simulink model "Huang_Isoherranen_Mechanistic_Kidney_Model"  (R2017b)
settings: Solver=VariableStepAuto  StartTime=0.0  StopTime=Tfinish  RelTol=1e-3  EnableMultiTasking=on
values from neighbouring files (symbols this model uses):
  alpha_1 = 1    [Huang_Isoherranen_Mechanistic_Kidney_Model_Example_Code.m]
  alpha_10 = 1    [Huang_Isoherranen_Mechanistic_Kidney_Model_Example_Code.m]
  alpha_11 = 1    [Huang_Isoherranen_Mechanistic_Kidney_Model_Example_Code.m]
  alpha_2 = 1    [Huang_Isoherranen_Mechanistic_Kidney_Model_Example_Code.m]
  alpha_3 = 1    [Huang_Isoherranen_Mechanistic_Kidney_Model_Example_Code.m]
  alpha_4 = 1    [Huang_Isoherranen_Mechanistic_Kidney_Model_Example_Code.m]
  alpha_5 = 1    [Huang_Isoherranen_Mechanistic_Kidney_Model_Example_Code.m]
  alpha_6 = 1    [Huang_Isoherranen_Mechanistic_Kidney_Model_Example_Code.m]
  alpha_7 = 1    [Huang_Isoherranen_Mechanistic_Kidney_Model_Example_Code.m]
  alpha_8 = 1    [Huang_Isoherranen_Mechanistic_Kidney_Model_Example_Code.m]
  alpha_9 = 1    [Huang_Isoherranen_Mechanistic_Kidney_Model_Example_Code.m]
  beta = 1    [Huang_Isoherranen_Mechanistic_Kidney_Model_Example_Code.m]
  BP0 = 1    [Huang_Isoherranen_Mechanistic_Kidney_Model_Example_Code.m]
  CL_api_reabs = 0    [Huang_Isoherranen_Mechanistic_Kidney_Model_Example_Code.m]
  CL_BC = 0    [Huang_Isoherranen_Mechanistic_Kidney_Model_Example_Code.m]
  CL_bsl_reabs = 0    [Huang_Isoherranen_Mechanistic_Kidney_Model_Example_Code.m]
  CL_CT = 0    [Huang_Isoherranen_Mechanistic_Kidney_Model_Example_Code.m]
  CL_kidney_intrinsic = 0    [Huang_Isoherranen_Mechanistic_Kidney_Model_Example_Code.m]
  CL_PD_CD = S_CD * Papp    (= 0.01608)    [Huang_Isoherranen_Mechanistic_Kidney_Model_Example_Code.m]
  CL_PD_DS = S_DT * Papp    (= 0.3744)    [Huang_Isoherranen_Mechanistic_Kidney_Model_Example_Code.m]
  CL_PD_LH = S_HT * Papp    (= 0.1464)    [Huang_Isoherranen_Mechanistic_Kidney_Model_Example_Code.m]
  CL_PD_PX_apical = S_PT * Papp    (= 14.6568)    [Huang_Isoherranen_Mechanistic_Kidney_Model_Example_Code.m]
  CL_PD_PX_basolateral = S_PT/30 * Papp    (= 0.48856)    [Huang_Isoherranen_Mechanistic_Kidney_Model_Example_Code.m]
  CLh = 0    [Huang_Isoherranen_Mechanistic_Kidney_Model_Example_Code.m]
  fu0 = 1    [Huang_Isoherranen_Mechanistic_Kidney_Model_Example_Code.m]
  fu_k = fu0    (= 1)    [Huang_Isoherranen_Mechanistic_Kidney_Model_Example_Code.m]
  gamma = 1    [Huang_Isoherranen_Mechanistic_Kidney_Model_Example_Code.m]
  Infusion_length = 240    [Huang_Isoherranen_Mechanistic_Kidney_Model_Example_Code.m]
  IR = 1    [Huang_Isoherranen_Mechanistic_Kidney_Model_Example_Code.m]
  ivbolusDose1 = 0    [Huang_Isoherranen_Mechanistic_Kidney_Model_Example_Code.m]
  ivT1 = 0    [Huang_Isoherranen_Mechanistic_Kidney_Model_Example_Code.m]
  Q_connectingtubule = 11    [Huang_Isoherranen_Mechanistic_Kidney_Model_Example_Code.m]
  Q_corticalCD = 7    [Huang_Isoherranen_Mechanistic_Kidney_Model_Example_Code.m]
  Q_GFR = 7.2    [Huang_Isoherranen_Mechanistic_Kidney_Model_Example_Code.m]
  Q_initialCD = 9    [Huang_Isoherranen_Mechanistic_Kidney_Model_Example_Code.m]
  Q_kidney0 = 60    [Huang_Isoherranen_Mechanistic_Kidney_Model_Example_Code.m]
  Q_medullaryCD = 5    [Huang_Isoherranen_Mechanistic_Kidney_Model_Example_Code.m]
  Q_papillary = 3    [Huang_Isoherranen_Mechanistic_Kidney_Model_Example_Code.m]
  Q_urine = 1    [Huang_Isoherranen_Mechanistic_Kidney_Model_Example_Code.m]
  Qc0 = 330    [Huang_Isoherranen_Mechanistic_Kidney_Model_Example_Code.m]
  Tstart_infusion = 0    [Huang_Isoherranen_Mechanistic_Kidney_Model_Example_Code.m]
  V_CDB = 0.237    [Huang_Isoherranen_Mechanistic_Kidney_Model_Example_Code.m]
  V_CDC = 0.237    [Huang_Isoherranen_Mechanistic_Kidney_Model_Example_Code.m]
  V_CDT = 0.237    [Huang_Isoherranen_Mechanistic_Kidney_Model_Example_Code.m]
  V_DB = 0.0194    [Huang_Isoherranen_Mechanistic_Kidney_Model_Example_Code.m]
  V_DC = 0.0194    [Huang_Isoherranen_Mechanistic_Kidney_Model_Example_Code.m]
  V_DT = 0.0194    [Huang_Isoherranen_Mechanistic_Kidney_Model_Example_Code.m]
  V_HB = 0.0027    [Huang_Isoherranen_Mechanistic_Kidney_Model_Example_Code.m]
  V_HC = 0.0027    [Huang_Isoherranen_Mechanistic_Kidney_Model_Example_Code.m]
  V_HT = 0.0027    [Huang_Isoherranen_Mechanistic_Kidney_Model_Example_Code.m]
  V_PB = 0.0305    [Huang_Isoherranen_Mechanistic_Kidney_Model_Example_Code.m]
  V_PC = 0.0305    [Huang_Isoherranen_Mechanistic_Kidney_Model_Example_Code.m]
  V_PT = 0.0305    [Huang_Isoherranen_Mechanistic_Kidney_Model_Example_Code.m]
  V_ven0 = 42    [Huang_Isoherranen_Mechanistic_Kidney_Model_Example_Code.m]
libraries: simulink x3, dspmathops x1
(part 2 of 2)

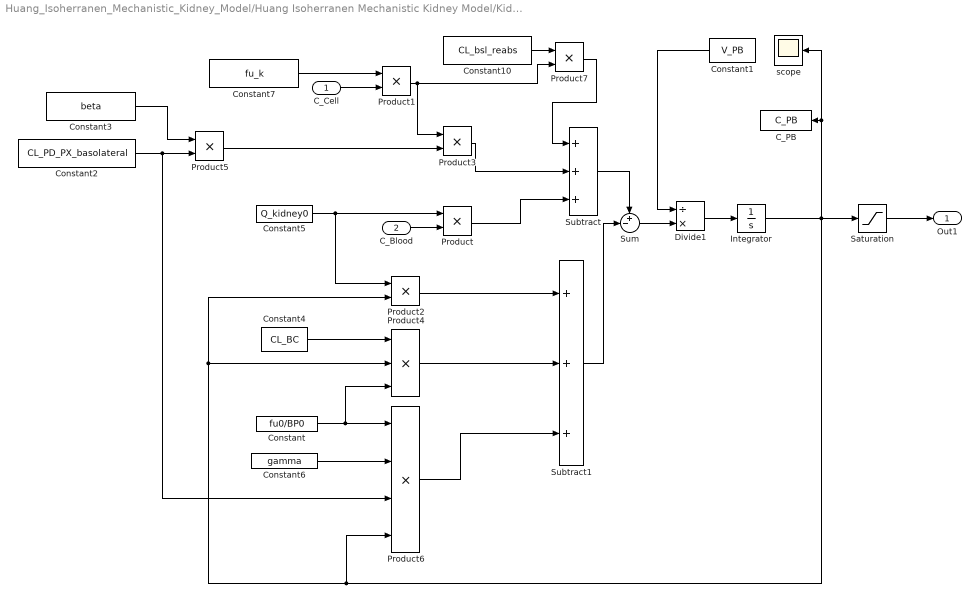
== system Huang_Isoherranen_Mechanistic_Kidney_Model/Huang Isoherranen Mechanistic Kidney Model/Kidney/Proximal blood ==
  C_Cell : Inport
  C_Blood : Inport  Port=2
  C_PB : ToWorkspace  VariableName=C_PB  SampleTime=-1
  Constant : Constant  Value=fu0/BP0
  Constant1 : Constant  Value=V_PB
  Constant10 : Constant  Value=CL_bsl_reabs
  Constant2 : Constant  Value=CL_PD_PX_basolateral
  Constant3 : Constant  Value=beta
  Constant4 : Constant  Value=CL_BC
  Constant5 : Constant  Value=Q_kidney0
  Constant6 : Constant  Value=gamma
  Constant7 : Constant  Value=fu_k
  Divide1 : Product  Inputs=/*
  Integrator : Integrator
  Product{,1..3,5,7} (6 alike) : Product  RndMeth=Zero
  Product4 : Product  Inputs=3  RndMeth=Zero
  Product6 : Product  Inputs=4  RndMeth=Zero
  Saturation : Saturate  UpperLimit=1000000000  LowerLimit=0
  Subtract : Sum  Inputs=+++
  Subtract1 : Sum  Inputs=+++
  Sum : Sum  Inputs=+-|
  scope : Scope
  Out1 : Outport
  wires:
  Integrator/1 -> Product6/4, Product2/2, Product4/2, Saturation/1, scope/1, C_PB/1
  Sum/1 -> Divide1/2
  Saturation/1 -> Out1/1
  Constant7/1 -> Product1/1
  Product1/1 -> Product3/1, Product7/2
  Constant5/1 -> Product2/1, Product/1
  Product3/1 -> Subtract/2
  Product/1 -> Subtract/3
  Constant1/1 -> Divide1/1
  Subtract/1 -> Sum/1
  Divide1/1 -> Integrator/1
  Constant3/1 -> Product5/1
  Constant2/1 -> Product6/3, Product5/2
  Product5/1 -> Product3/2
  Subtract1/1 -> Sum/2
  C_Cell/1 -> Product1/2
  C_Blood/1 -> Product/2
  Constant/1 -> Product4/3, Product6/1
  Product2/1 -> Subtract1/1
  Constant6/1 -> Product6/2
  Product6/1 -> Subtract1/3
  Constant4/1 -> Product4/1
  Product4/1 -> Subtract1/2
  Constant10/1 -> Product7/1
  Product7/1 -> Subtract/1

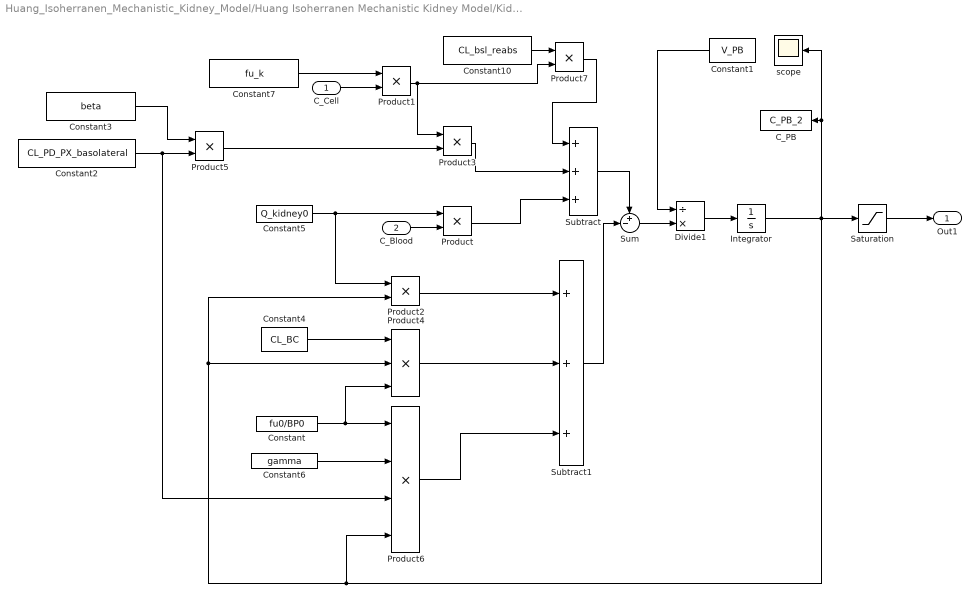
== system Huang_Isoherranen_Mechanistic_Kidney_Model/Huang Isoherranen Mechanistic Kidney Model/Kidney/Proximal blood1 ==
  C_Cell : Inport
  C_Blood : Inport  Port=2
  C_PB : ToWorkspace  VariableName=C_PB_2  SampleTime=-1
  Constant : Constant  Value=fu0/BP0
  Constant1 : Constant  Value=V_PB
  Constant10 : Constant  Value=CL_bsl_reabs
  Constant2 : Constant  Value=CL_PD_PX_basolateral
  Constant3 : Constant  Value=beta
  Constant4 : Constant  Value=CL_BC
  Constant5 : Constant  Value=Q_kidney0
  Constant6 : Constant  Value=gamma
  Constant7 : Constant  Value=fu_k
  Divide1 : Product  Inputs=/*
  Integrator : Integrator
  Product{,1..3,5,7} (6 alike) : Product  RndMeth=Zero
  Product4 : Product  Inputs=3  RndMeth=Zero
  Product6 : Product  Inputs=4  RndMeth=Zero
  Saturation : Saturate  UpperLimit=1000000000  LowerLimit=0
  Subtract : Sum  Inputs=+++
  Subtract1 : Sum  Inputs=+++
  Sum : Sum  Inputs=+-|
  scope : Scope
  Out1 : Outport
  wires:
  Integrator/1 -> Product6/4, Product2/2, Product4/2, Saturation/1, scope/1, C_PB/1
  Sum/1 -> Divide1/2
  Saturation/1 -> Out1/1
  Constant7/1 -> Product1/1
  Product1/1 -> Product3/1, Product7/2
  Constant5/1 -> Product2/1, Product/1
  Product3/1 -> Subtract/2
  Product/1 -> Subtract/3
  Constant1/1 -> Divide1/1
  Subtract/1 -> Sum/1
  Divide1/1 -> Integrator/1
  Constant3/1 -> Product5/1
  Constant2/1 -> Product6/3, Product5/2
  Product5/1 -> Product3/2
  Subtract1/1 -> Sum/2
  C_Cell/1 -> Product1/2
  C_Blood/1 -> Product/2
  Constant/1 -> Product4/3, Product6/1
  Product2/1 -> Subtract1/1
  Constant6/1 -> Product6/2
  Product6/1 -> Subtract1/3
  Constant4/1 -> Product4/1
  Product4/1 -> Subtract1/2
  Constant10/1 -> Product7/1
  Product7/1 -> Subtract/1

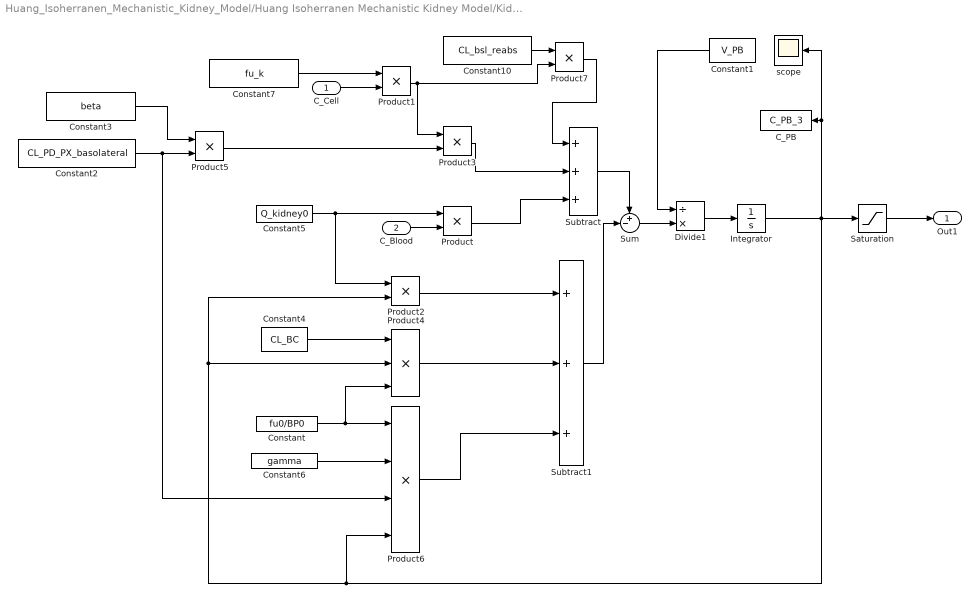
== system Huang_Isoherranen_Mechanistic_Kidney_Model/Huang Isoherranen Mechanistic Kidney Model/Kidney/Proximal blood2 ==
  C_Cell : Inport
  C_Blood : Inport  Port=2
  C_PB : ToWorkspace  VariableName=C_PB_3  SampleTime=-1
  Constant : Constant  Value=fu0/BP0
  Constant1 : Constant  Value=V_PB
  Constant10 : Constant  Value=CL_bsl_reabs
  Constant2 : Constant  Value=CL_PD_PX_basolateral
  Constant3 : Constant  Value=beta
  Constant4 : Constant  Value=CL_BC
  Constant5 : Constant  Value=Q_kidney0
  Constant6 : Constant  Value=gamma
  Constant7 : Constant  Value=fu_k
  Divide1 : Product  Inputs=/*
  Integrator : Integrator
  Product{,1..3,5,7} (6 alike) : Product  RndMeth=Zero
  Product4 : Product  Inputs=3  RndMeth=Zero
  Product6 : Product  Inputs=4  RndMeth=Zero
  Saturation : Saturate  UpperLimit=1000000000  LowerLimit=0
  Subtract : Sum  Inputs=+++
  Subtract1 : Sum  Inputs=+++
  Sum : Sum  Inputs=+-|
  scope : Scope
  Out1 : Outport
  wires:
  Integrator/1 -> Product6/4, Product2/2, Product4/2, Saturation/1, scope/1, C_PB/1
  Sum/1 -> Divide1/2
  Saturation/1 -> Out1/1
  Constant7/1 -> Product1/1
  Product1/1 -> Product3/1, Product7/2
  Constant5/1 -> Product2/1, Product/1
  Product3/1 -> Subtract/2
  Product/1 -> Subtract/3
  Constant1/1 -> Divide1/1
  Subtract/1 -> Sum/1
  Divide1/1 -> Integrator/1
  Constant3/1 -> Product5/1
  Constant2/1 -> Product6/3, Product5/2
  Product5/1 -> Product3/2
  Subtract1/1 -> Sum/2
  C_Cell/1 -> Product1/2
  C_Blood/1 -> Product/2
  Constant/1 -> Product4/3, Product6/1
  Product2/1 -> Subtract1/1
  Constant6/1 -> Product6/2
  Product6/1 -> Subtract1/3
  Constant4/1 -> Product4/1
  Product4/1 -> Subtract1/2
  Constant10/1 -> Product7/1
  Product7/1 -> Subtract/1

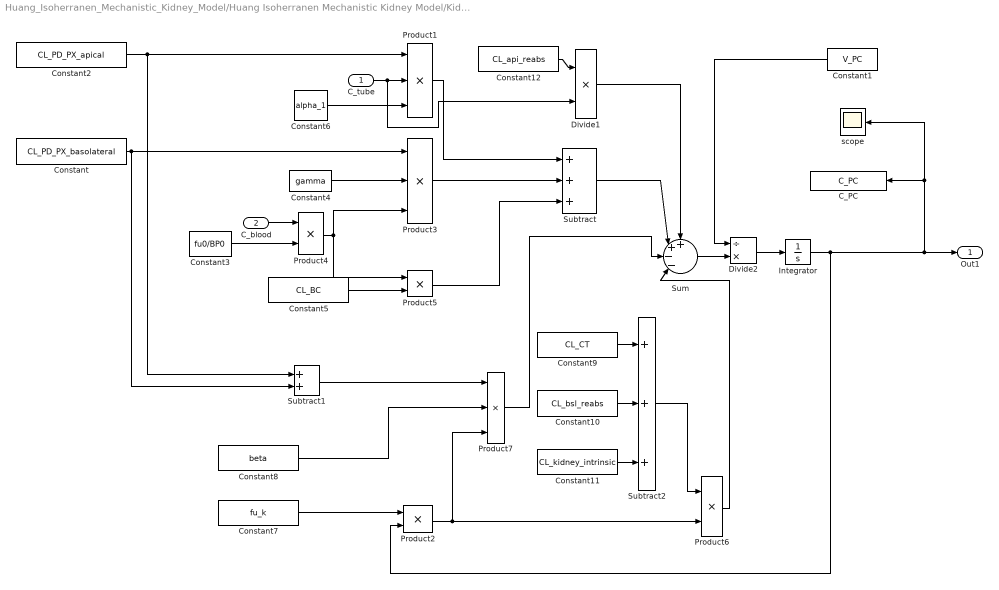
== system Huang_Isoherranen_Mechanistic_Kidney_Model/Huang Isoherranen Mechanistic Kidney Model/Kidney/Proximal cell ==
  C_tube : Inport
  C_blood : Inport  Port=2
  C_PC : ToWorkspace  VariableName=C_PC  SampleTime=-1
  Constant : Constant  Value=CL_PD_PX_basolateral
  Constant1 : Constant  Value=V_PC
  Constant10 : Constant  Value=CL_bsl_reabs
  Constant11 : Constant  Value=CL_kidney_intrinsic
  Constant12 : Constant  Value=CL_api_reabs
  Constant2 : Constant  Value=CL_PD_PX_apical
  Constant3 : Constant  Value=fu0/BP0
  Constant4 : Constant  Value=gamma
  Constant5 : Constant  Value=CL_BC
  Constant6 : Constant  Value=alpha_1
  Constant7 : Constant  Value=fu_k
  Constant8 : Constant  Value=beta
  Constant9 : Constant  Value=CL_CT
  Divide1 : Product  Inputs=**
  Divide2 : Product  Inputs=/*
  Integrator : Integrator
  Product1 : Product  Inputs=3  RndMeth=Zero
  Product{2,4..6} (4 alike) : Product  RndMeth=Zero
  Product3 : Product  Inputs=3  RndMeth=Zero
  Product7 : Product  Inputs=3  RndMeth=Zero
  Subtract : Sum  Inputs=+++
  Subtract1 : Sum
  Subtract2 : Sum  Inputs=+++
  Sum : Sum  Inputs=++--|
  scope : Scope
  Out1 : Outport
  wires:
  Integrator/1 -> Product2/2, Out1/1, scope/1, C_PC/1
  C_tube/1 -> Divide1/2, Product1/2
  Constant2/1 -> Subtract1/1, Product1/1
  Constant4/1 -> Product3/2
  Subtract/1 -> Sum/2
  Product3/1 -> Subtract/2
  C_blood/1 -> Product4/1
  Constant3/1 -> Product4/2
  Product4/1 -> Product5/1, Product3/3
  Constant5/1 -> Product5/2
  Constant6/1 -> Product1/3
  Product5/1 -> Subtract/3
  Product1/1 -> Subtract/1
  Sum/1 -> Divide2/2
  Constant1/1 -> Divide2/1
  Divide2/1 -> Integrator/1
  Product2/1 -> Product6/2, Product7/3
  Constant7/1 -> Product2/1
  Constant8/1 -> Product7/2
  Product6/1 -> Sum/4
  Product7/1 -> Sum/3
  Subtract1/1 -> Product7/1
  Constant/1 -> Subtract1/2, Product3/1
  Constant12/1 -> Divide1/1
  Divide1/1 -> Sum/1
  Constant10/1 -> Subtract2/2
  Subtract2/1 -> Product6/1
  Constant9/1 -> Subtract2/1
  Constant11/1 -> Subtract2/3

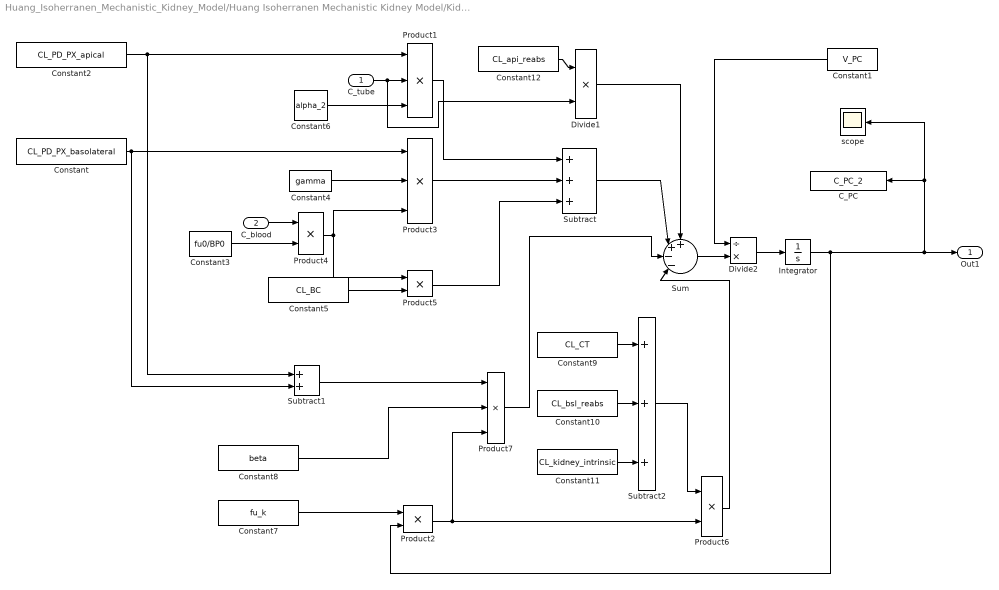
== system Huang_Isoherranen_Mechanistic_Kidney_Model/Huang Isoherranen Mechanistic Kidney Model/Kidney/Proximal cell1 ==
  C_tube : Inport
  C_blood : Inport  Port=2
  C_PC : ToWorkspace  VariableName=C_PC_2  SampleTime=-1
  Constant : Constant  Value=CL_PD_PX_basolateral
  Constant1 : Constant  Value=V_PC
  Constant10 : Constant  Value=CL_bsl_reabs
  Constant11 : Constant  Value=CL_kidney_intrinsic
  Constant12 : Constant  Value=CL_api_reabs
  Constant2 : Constant  Value=CL_PD_PX_apical
  Constant3 : Constant  Value=fu0/BP0
  Constant4 : Constant  Value=gamma
  Constant5 : Constant  Value=CL_BC
  Constant6 : Constant  Value=alpha_2
  Constant7 : Constant  Value=fu_k
  Constant8 : Constant  Value=beta
  Constant9 : Constant  Value=CL_CT
  Divide1 : Product  Inputs=**
  Divide2 : Product  Inputs=/*
  Integrator : Integrator
  Product1 : Product  Inputs=3  RndMeth=Zero
  Product{2,4..6} (4 alike) : Product  RndMeth=Zero
  Product3 : Product  Inputs=3  RndMeth=Zero
  Product7 : Product  Inputs=3  RndMeth=Zero
  Subtract : Sum  Inputs=+++
  Subtract1 : Sum
  Subtract2 : Sum  Inputs=+++
  Sum : Sum  Inputs=++--|
  scope : Scope
  Out1 : Outport
  wires:
  Integrator/1 -> Product2/2, Out1/1, scope/1, C_PC/1
  C_tube/1 -> Divide1/2, Product1/2
  Constant2/1 -> Subtract1/1, Product1/1
  Constant4/1 -> Product3/2
  Subtract/1 -> Sum/2
  Product3/1 -> Subtract/2
  C_blood/1 -> Product4/1
  Constant3/1 -> Product4/2
  Product4/1 -> Product5/1, Product3/3
  Constant5/1 -> Product5/2
  Constant6/1 -> Product1/3
  Product5/1 -> Subtract/3
  Product1/1 -> Subtract/1
  Sum/1 -> Divide2/2
  Constant1/1 -> Divide2/1
  Divide2/1 -> Integrator/1
  Product2/1 -> Product6/2, Product7/3
  Constant7/1 -> Product2/1
  Constant8/1 -> Product7/2
  Product6/1 -> Sum/4
  Product7/1 -> Sum/3
  Subtract1/1 -> Product7/1
  Constant/1 -> Subtract1/2, Product3/1
  Constant12/1 -> Divide1/1
  Divide1/1 -> Sum/1
  Constant10/1 -> Subtract2/2
  Subtract2/1 -> Product6/1
  Constant9/1 -> Subtract2/1
  Constant11/1 -> Subtract2/3

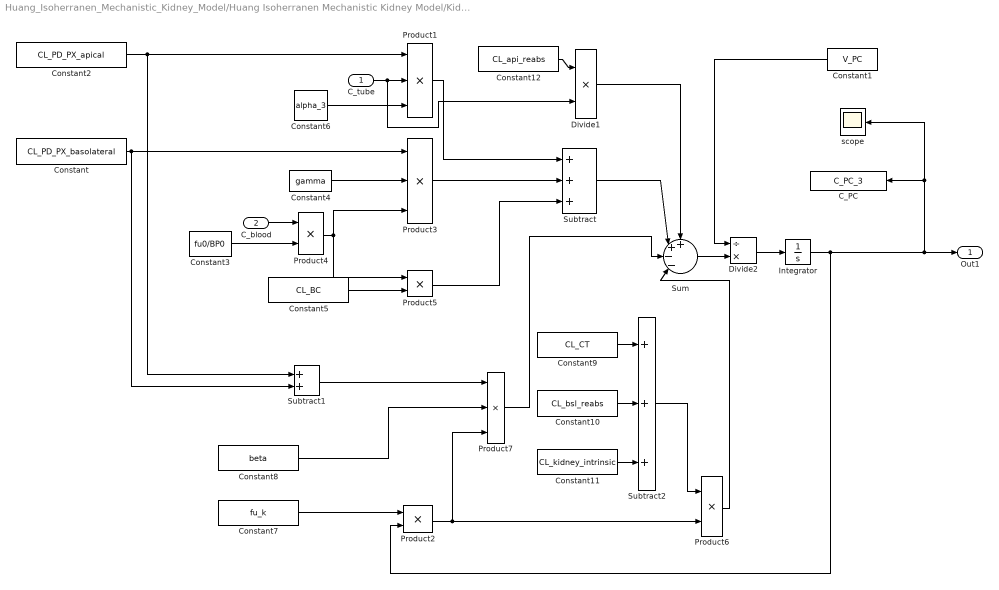
== system Huang_Isoherranen_Mechanistic_Kidney_Model/Huang Isoherranen Mechanistic Kidney Model/Kidney/Proximal cell2 ==
  C_tube : Inport
  C_blood : Inport  Port=2
  C_PC : ToWorkspace  VariableName=C_PC_3  SampleTime=-1
  Constant : Constant  Value=CL_PD_PX_basolateral
  Constant1 : Constant  Value=V_PC
  Constant10 : Constant  Value=CL_bsl_reabs
  Constant11 : Constant  Value=CL_kidney_intrinsic
  Constant12 : Constant  Value=CL_api_reabs
  Constant2 : Constant  Value=CL_PD_PX_apical
  Constant3 : Constant  Value=fu0/BP0
  Constant4 : Constant  Value=gamma
  Constant5 : Constant  Value=CL_BC
  Constant6 : Constant  Value=alpha_3
  Constant7 : Constant  Value=fu_k
  Constant8 : Constant  Value=beta
  Constant9 : Constant  Value=CL_CT
  Divide1 : Product  Inputs=**
  Divide2 : Product  Inputs=/*
  Integrator : Integrator
  Product1 : Product  Inputs=3  RndMeth=Zero
  Product{2,4..6} (4 alike) : Product  RndMeth=Zero
  Product3 : Product  Inputs=3  RndMeth=Zero
  Product7 : Product  Inputs=3  RndMeth=Zero
  Subtract : Sum  Inputs=+++
  Subtract1 : Sum
  Subtract2 : Sum  Inputs=+++
  Sum : Sum  Inputs=++--|
  scope : Scope
  Out1 : Outport
  wires:
  Integrator/1 -> Product2/2, Out1/1, scope/1, C_PC/1
  C_tube/1 -> Divide1/2, Product1/2
  Constant2/1 -> Subtract1/1, Product1/1
  Constant4/1 -> Product3/2
  Subtract/1 -> Sum/2
  Product3/1 -> Subtract/2
  C_blood/1 -> Product4/1
  Constant3/1 -> Product4/2
  Product4/1 -> Product5/1, Product3/3
  Constant5/1 -> Product5/2
  Constant6/1 -> Product1/3
  Product5/1 -> Subtract/3
  Product1/1 -> Subtract/1
  Sum/1 -> Divide2/2
  Constant1/1 -> Divide2/1
  Divide2/1 -> Integrator/1
  Product2/1 -> Product6/2, Product7/3
  Constant7/1 -> Product2/1
  Constant8/1 -> Product7/2
  Product6/1 -> Sum/4
  Product7/1 -> Sum/3
  Subtract1/1 -> Product7/1
  Constant/1 -> Subtract1/2, Product3/1
  Constant12/1 -> Divide1/1
  Divide1/1 -> Sum/1
  Constant10/1 -> Subtract2/2
  Subtract2/1 -> Product6/1
  Constant9/1 -> Subtract2/1
  Constant11/1 -> Subtract2/3

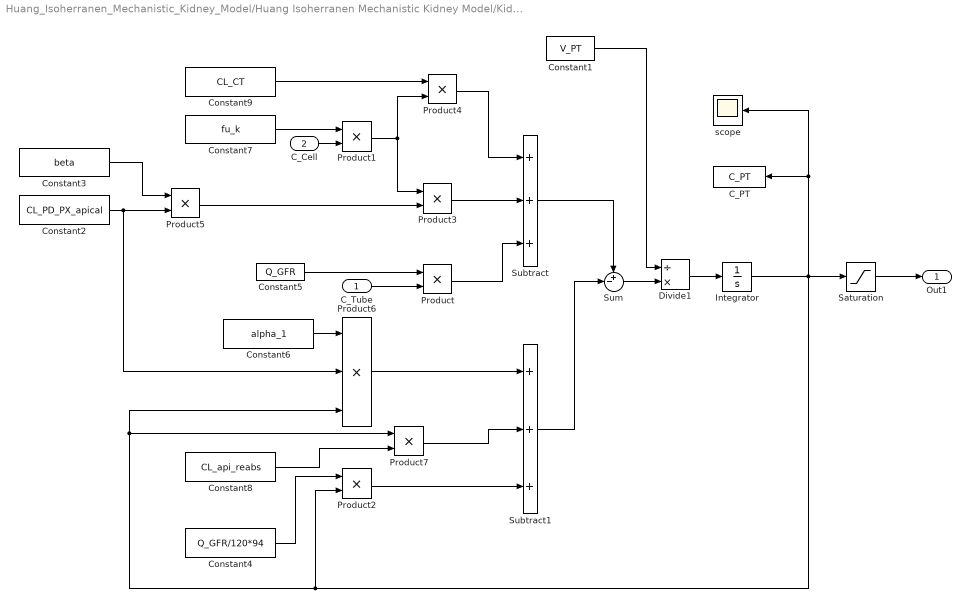
== system Huang_Isoherranen_Mechanistic_Kidney_Model/Huang Isoherranen Mechanistic Kidney Model/Kidney/Proximal tube ==
  C_Tube : Inport
  C_Cell : Inport  Port=2
  C_PT : ToWorkspace  VariableName=C_PT  SampleTime=-1
  Constant1 : Constant  Value=V_PT
  Constant2 : Constant  Value=CL_PD_PX_apical
  Constant3 : Constant  Value=beta
  Constant4 : Constant  Value=Q_GFR/120*94
  Constant5 : Constant  Value=Q_GFR
  Constant6 : Constant  Value=alpha_1
  Constant7 : Constant  Value=fu_k
  Constant8 : Constant  Value=CL_api_reabs
  Constant9 : Constant  Value=CL_CT
  Divide1 : Product  Inputs=/*
  Integrator : Integrator
  Product{,1..5,7} (7 alike) : Product  RndMeth=Zero
  Product6 : Product  Inputs=3  RndMeth=Zero
  Saturation : Saturate  UpperLimit=1000000000  LowerLimit=0
  Subtract : Sum  Inputs=+++
  Subtract1 : Sum  Inputs=+++
  Sum : Sum  Inputs=+-|
  scope : Scope
  Out1 : Outport
  wires:
  Integrator/1 -> Product2/2, Product6/3, Product7/1, Saturation/1, scope/1, C_PT/1
  Sum/1 -> Divide1/2
  Saturation/1 -> Out1/1
  C_Tube/1 -> Product/2
  Constant7/1 -> Product1/1
  C_Cell/1 -> Product1/2
  Product1/1 -> Product3/1, Product4/2
  Constant5/1 -> Product/1
  Product4/1 -> Subtract/1
  Product3/1 -> Subtract/2
  Product/1 -> Subtract/3
  Constant1/1 -> Divide1/1
  Subtract/1 -> Sum/1
  Divide1/1 -> Integrator/1
  Constant4/1 -> Product2/1
  Constant3/1 -> Product5/1
  Constant2/1 -> Product6/2, Product5/2
  Constant9/1 -> Product4/1
  Product5/1 -> Product3/2
  Constant6/1 -> Product6/1
  Product6/1 -> Subtract1/1
  Product2/1 -> Subtract1/3
  Subtract1/1 -> Sum/2
  Product7/1 -> Subtract1/2
  Constant8/1 -> Product7/2

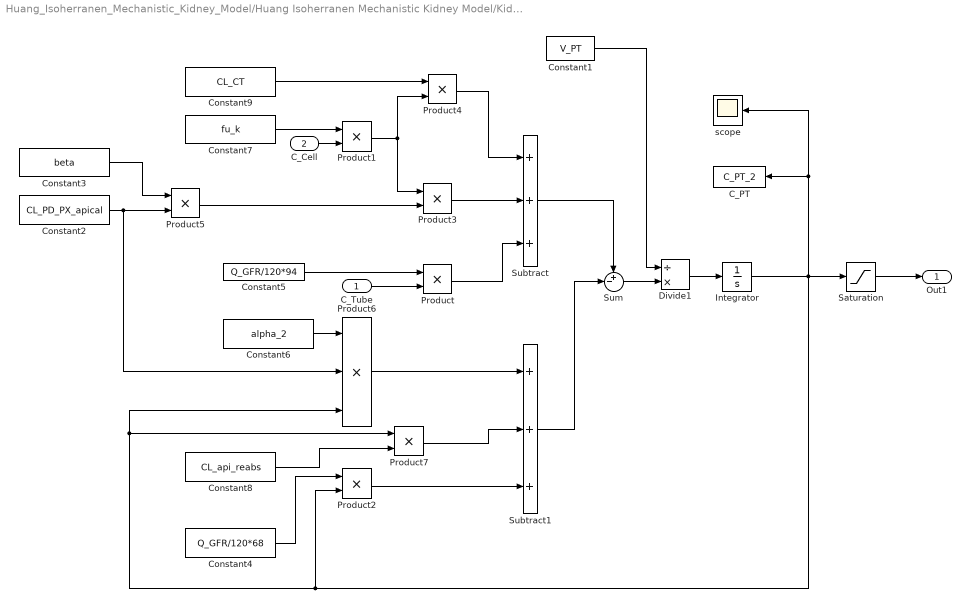
== system Huang_Isoherranen_Mechanistic_Kidney_Model/Huang Isoherranen Mechanistic Kidney Model/Kidney/Proximal tube1 ==
  C_Tube : Inport
  C_Cell : Inport  Port=2
  C_PT : ToWorkspace  VariableName=C_PT_2  SampleTime=-1
  Constant1 : Constant  Value=V_PT
  Constant2 : Constant  Value=CL_PD_PX_apical
  Constant3 : Constant  Value=beta
  Constant4 : Constant  Value=Q_GFR/120*68
  Constant5 : Constant  Value=Q_GFR/120*94
  Constant6 : Constant  Value=alpha_2
  Constant7 : Constant  Value=fu_k
  Constant8 : Constant  Value=CL_api_reabs
  Constant9 : Constant  Value=CL_CT
  Divide1 : Product  Inputs=/*
  Integrator : Integrator
  Product{,1..5,7} (7 alike) : Product  RndMeth=Zero
  Product6 : Product  Inputs=3  RndMeth=Zero
  Saturation : Saturate  UpperLimit=1000000000  LowerLimit=0
  Subtract : Sum  Inputs=+++
  Subtract1 : Sum  Inputs=+++
  Sum : Sum  Inputs=+-|
  scope : Scope
  Out1 : Outport
  wires:
  Integrator/1 -> Product2/2, Product6/3, Product7/1, Saturation/1, scope/1, C_PT/1
  Sum/1 -> Divide1/2
  Saturation/1 -> Out1/1
  C_Tube/1 -> Product/2
  Constant7/1 -> Product1/1
  C_Cell/1 -> Product1/2
  Product1/1 -> Product3/1, Product4/2
  Constant5/1 -> Product/1
  Product4/1 -> Subtract/1
  Product3/1 -> Subtract/2
  Product/1 -> Subtract/3
  Constant1/1 -> Divide1/1
  Subtract/1 -> Sum/1
  Divide1/1 -> Integrator/1
  Constant4/1 -> Product2/1
  Constant3/1 -> Product5/1
  Constant2/1 -> Product6/2, Product5/2
  Constant9/1 -> Product4/1
  Product5/1 -> Product3/2
  Constant6/1 -> Product6/1
  Product6/1 -> Subtract1/1
  Product2/1 -> Subtract1/3
  Subtract1/1 -> Sum/2
  Product7/1 -> Subtract1/2
  Constant8/1 -> Product7/2

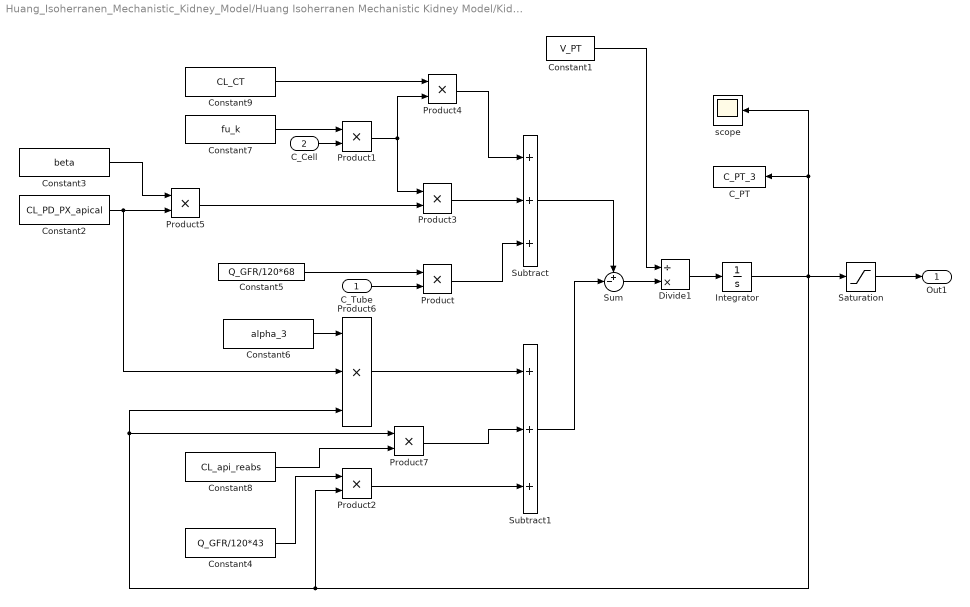
== system Huang_Isoherranen_Mechanistic_Kidney_Model/Huang Isoherranen Mechanistic Kidney Model/Kidney/Proximal tube2 ==
  C_Tube : Inport
  C_Cell : Inport  Port=2
  C_PT : ToWorkspace  VariableName=C_PT_3  SampleTime=-1
  Constant1 : Constant  Value=V_PT
  Constant2 : Constant  Value=CL_PD_PX_apical
  Constant3 : Constant  Value=beta
  Constant4 : Constant  Value=Q_GFR/120*43
  Constant5 : Constant  Value=Q_GFR/120*68
  Constant6 : Constant  Value=alpha_3
  Constant7 : Constant  Value=fu_k
  Constant8 : Constant  Value=CL_api_reabs
  Constant9 : Constant  Value=CL_CT
  Divide1 : Product  Inputs=/*
  Integrator : Integrator
  Product{,1..5,7} (7 alike) : Product  RndMeth=Zero
  Product6 : Product  Inputs=3  RndMeth=Zero
  Saturation : Saturate  UpperLimit=1000000000  LowerLimit=0
  Subtract : Sum  Inputs=+++
  Subtract1 : Sum  Inputs=+++
  Sum : Sum  Inputs=+-|
  scope : Scope
  Out1 : Outport
  wires:
  Integrator/1 -> Product2/2, Product6/3, Product7/1, Saturation/1, scope/1, C_PT/1
  Sum/1 -> Divide1/2
  Saturation/1 -> Out1/1
  C_Tube/1 -> Product/2
  Constant7/1 -> Product1/1
  C_Cell/1 -> Product1/2
  Product1/1 -> Product3/1, Product4/2
  Constant5/1 -> Product/1
  Product4/1 -> Subtract/1
  Product3/1 -> Subtract/2
  Product/1 -> Subtract/3
  Constant1/1 -> Divide1/1
  Subtract/1 -> Sum/1
  Divide1/1 -> Integrator/1
  Constant4/1 -> Product2/1
  Constant3/1 -> Product5/1
  Constant2/1 -> Product6/2, Product5/2
  Constant9/1 -> Product4/1
  Product5/1 -> Product3/2
  Constant6/1 -> Product6/1
  Product6/1 -> Subtract1/1
  Product2/1 -> Subtract1/3
  Subtract1/1 -> Sum/2
  Product7/1 -> Subtract1/2
  Constant8/1 -> Product7/2

== system Huang_Isoherranen_Mechanistic_Kidney_Model/Huang Isoherranen Mechanistic Kidney Model/venous blood/IV Infusion1 ==
  In1 : Inport
  Add : Sum  Inputs=+-
  Clock1 : Clock
  Compare To Constant : simulink/Logic and Bit Operations/Compare To Constant  relop=>=  const=0  OutDataTypeStr=boolean
  Compare To Constant1 : simulink/Logic and Bit Operations/Compare To Constant  relop=<=  const=Infusion_length  OutDataTypeStr=boolean
  Constant1 : Constant
  Constant2 : Constant  Value=1/(V_ven0)
  Constant3 : Constant  Value=Qc0
  Constant4 : Constant  Value=1/Qc0
  Divide{5..8} (4 alike) : Product  Inputs=**
  Gain2 : Gain  Gain=-1
  Math Function1 : Math  SaturateOnIntegerOverflow=on
  Product1 : Product  RndMeth=Zero
  Product2 : Product  RndMeth=Zero
  poDose2 : Fcn  Expr=u(1)-Tstart_infusion
  Out1 : Outport
  wires:
  Clock1/1 -> poDose2/1
  Divide5/1 -> Divide6/1  "-Qc/V"
  Constant2/1 -> Divide5/1
  Gain2/1 -> Divide5/2
  poDose2/1 -> Compare To Constant/1, Product1/1
  Divide6/1 -> Math Function1/1
  In1/1 -> Divide7/1
  Math Function1/1 -> Add/2
  Constant1/1 -> Add/1
  Divide7/1 -> Divide8/2
  Divide8/1 -> Out1/1
  Constant4/1 -> Divide7/2
  Compare To Constant/1 -> Product1/2
  Add/1 -> Divide8/1
  Product1/1 -> Product2/1, Compare To Constant1/1
  Product2/1 -> Divide6/2
  Compare To Constant1/1 -> Product2/2
  Constant3/1 -> Gain2/1

== system Huang_Isoherranen_Mechanistic_Kidney_Model/Huang Isoherranen Mechanistic Kidney Model/venous blood/ivDose1 ==
  In1 : Inport
  Clock : Clock
  Compare To Zero : simulink/Logic and Bit Operations/Compare To Zero  relop=>=  OutDataTypeStr=uint8
  Constant : Constant
  Constant1 : Constant  Value=1/(V_ven0)
  Constant2 : Constant  Value=Qc0
  Divide : Product  Inputs=*/
  Divide{1..4} (4 alike) : Product  Inputs=**
  Gain1 : Gain  Gain=-1
  Math Function : Math  SaturateOnIntegerOverflow=on
  Product2 : Product  RndMeth=Zero
  Product3 : Product  RndMeth=Zero
  Scope : Scope
  To Workspace : ToWorkspace  VariableName=V_ven  SampleTime=-1
  iv_1 : Scope
  poDose1 : Fcn  Expr=u(1)-ivT1
  Out1 : Outport
  wires:
  Constant2/1 -> Gain1/1
  Gain1/1 -> Divide1/2
  Constant1/1 -> Divide/2, Divide1/1, Divide4/2
  Constant/1 -> Divide/1
  Divide/1 -> To Workspace/1, Scope/1
  poDose1/1 -> Compare To Zero/1, Product2/1
  Compare To Zero/1 -> Product2/2, Product3/2
  Clock/1 -> poDose1/1
  Product3/1 -> iv_1/1, Out1/1
  Divide1/1 -> Divide2/1  "-Qc/V"
  Product2/1 -> Divide2/2
  Divide2/1 -> Math Function/1
  Math Function/1 -> Divide3/2
  Divide3/1 -> Product3/1
  In1/1 -> Divide4/1
  Divide4/1 -> Divide3/1
